simulink subsystem "fcn_HVCellBalanceCheck"  (R2021b)
settings: Solver=VariableStepAuto  StartTime=0.0  StopTime=10.0  RelTol=1e-3
settings Model: Creator=SidharthUrbanMobilit  LastModifiedBy=AbulUrbanMobilitySys
settings SolverCC: AlgebraicLoopSolver=TrustRegion
settings DebuggingCC: SFMachineParentedDataDiag=warning

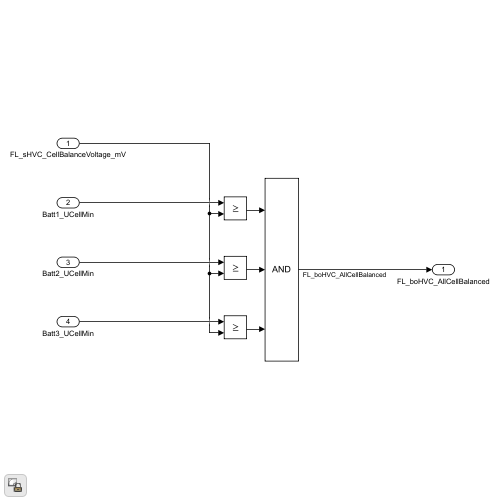
[thumbnail: Simulink's stored preview of the top-level diagram]
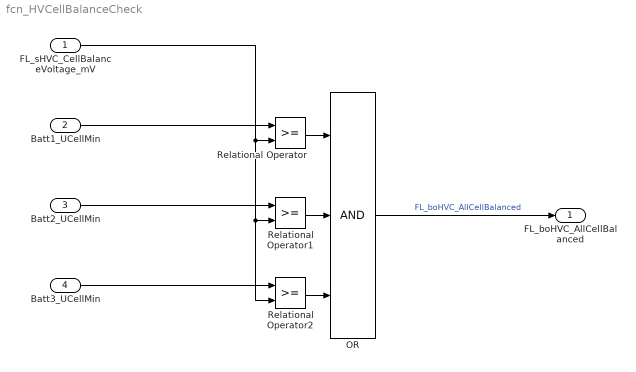
== system fcn_HVCellBalanceCheck ==
  FL_sHVC_CellBalanceVoltage_mV : Inport  OutDataTypeStr=single
  Batt1_UCellMin : Inport  Port=2  OutDataTypeStr=single
  Batt2_UCellMin : Inport  Port=3  OutDataTypeStr=single
  Batt3_UCellMin : Inport  Port=4  OutDataTypeStr=single
  OR : Logic  Inputs=3  AllPortsSameDT=off  OutDataTypeStr=boolean
  Relational Operator : RelationalOperator  OutDataTypeStr=boolean  RndMeth=Simplest
  Relational Operator1 : RelationalOperator  OutDataTypeStr=boolean  RndMeth=Simplest
  Relational Operator2 : RelationalOperator  OutDataTypeStr=boolean  RndMeth=Simplest
  FL_boHVC_AllCellBalanced : Outport  OutDataTypeStr=boolean
  wires:
  Batt3_UCellMin/1 -> Relational Operator2/1
  Batt1_UCellMin/1 -> Relational Operator/1
  OR/1 -> FL_boHVC_AllCellBalanced/1  "FL_boHVC_AllCellBalanced"
  Relational Operator1/1 -> OR/2
  Batt2_UCellMin/1 -> Relational Operator1/1
  FL_sHVC_CellBalanceVoltage_mV/1 -> Relational Operator2/2, Relational Operator1/2, Relational Operator/2
  Relational Operator2/1 -> OR/3
  Relational Operator/1 -> OR/1
